simulink model "massMatrix"  (R2017b)
settings: Solver=VariableStepAuto  StartTime=0.0  StopTime=10.0  RelTol=1e-3
settings Model: Creator=guoro  LastModifiedBy=guoro

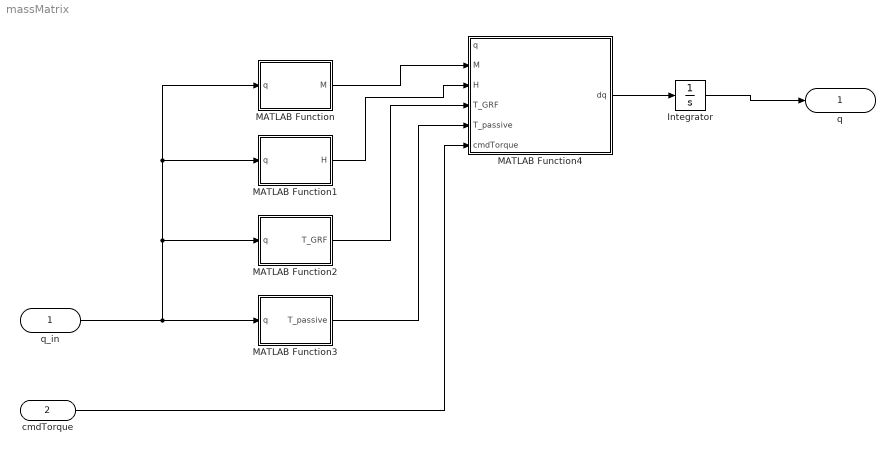
== system massMatrix ==
  "q_in " : Inport
  cmdTorque : Inport  Port=2
  Integrator : Integrator
  MATLAB Function : MATLAB Function  TreatAsAtomicUnit=on
  MATLAB Function1 : MATLAB Function  TreatAsAtomicUnit=on
  MATLAB Function2 : MATLAB Function  TreatAsAtomicUnit=on
  MATLAB Function3 : MATLAB Function  TreatAsAtomicUnit=on
  MATLAB Function4 : MATLAB Function  TreatAsAtomicUnit=on
  q : Outport
  wires:
  MATLAB Function/1(M) -> MATLAB Function4/2(M)
  MATLAB Function1/1(H) -> MATLAB Function4/3(H)
  MATLAB Function2/1(T_GRF) -> MATLAB Function4/4(T_GRF)
  MATLAB Function3/1(T_passive) -> MATLAB Function4/5(T_passive)
  MATLAB Function4/1(dq) -> Integrator/1
  Integrator/1 -> q/1
  cmdTorque/1 -> MATLAB Function4/6(cmdTorque)
  "q_in "/1 -> MATLAB Function1/1(q), MATLAB Function/1(q), MATLAB Function2/1(q), MATLAB Function3/1(q)

== matlab function massMatrix/MATLAB Function1 ==
  data: q input; H output
function H = coriolisTerm(q)
    H = [49.05  * cos(q(1)) - 6.13125 * cos(q(1)) * cos(q(2)) + 6.13125 * sin(q(1)) * sin(q(2)) + 0.625 * sin(q(2)) * q(3) * q(4) + 0.3125 * sin(q(2)) * q(4)^2;
         -6.13125 * cos(q(1)) * cos(q(2)) + 6.13125 * sin(q(1)) * sin(q(2)) - 0.3125 * sin(q(2)) * q(3)^2];
end

== matlab function massMatrix/MATLAB Function ==
  data: q input; M output
function M = massMatrix(q)
 %% Lagrange-Euler Method : Mass Matrix
 M = [2.1875 - 0.625 * cos(q(2)), 0.104167 - 0.3125 * cos(q(2)); 0.104167-0.3125 * cos(q(2)), 0.104167];
end

== matlab function massMatrix/MATLAB Function2 ==
  data: q input; T_GRF output
function T_GRF = groundRForce(q)
    T_GRF = [0; 0];
end

== matlab function massMatrix/MATLAB Function3 ==
  data: q input; T_passive output
function T_passive = passiveJoint(q)
    % Passive Joint Constants
    Ks = 30;
    Bs = 10;
    theta_eq = 2/3 * pi;

    T_passive = [0; -Ks * (q(1) - theta_eq) - Bs * q(4)];
end

== matlab function massMatrix/MATLAB Function4 ==
  data: q input; dq output; M input; H input; T_GRF input; T_passive input; cmdTorque input
function dq = InverseDynamics(q, M, H, T_GRF, T_passive, cmdTorque)
    dq = zeros(4, 1);
    dq(1:2) = q(3:4);
    dq(3:4) = M\(-H + T_GRF + T_passive + cmdTorque);
end
